simulink model "Gates"  (R2024b)
settings: Solver=FixedStepAuto  StartTime=0  StopTime=1  FixedStep=0.00001  RelTol=1e-3
libraries: spsTriangleGeneratorLib x1
(part 2 of 2)

== system Gates/Subsystem5/Adder & Logic Module/Subsystem6 ==
  Carry In : Inport
  = So far : Inport  Port=2
  A>B Prev : Inport  Port=3
  B : Inport  Port=4
  A : Inport  Port=5
  Subtract : Inport  Port=6
  AND : Logic  IconShape=distinctive  AllPortsSameDT=off  OutDataTypeStr=boolean
  AND1 : Logic  IconShape=distinctive  AllPortsSameDT=off  OutDataTypeStr=boolean
  AND2 : Logic  IconShape=distinctive  AllPortsSameDT=off  OutDataTypeStr=boolean
  AND3 : Logic  Inputs=3  IconShape=distinctive  AllPortsSameDT=off  OutDataTypeStr=boolean
  Mux : Mux  Inputs=6
  NOT : Logic  Operator=NOT  IconShape=distinctive  AllPortsSameDT=off  OutDataTypeStr=boolean
  NOT1 : Logic  Operator=NOT  IconShape=distinctive  AllPortsSameDT=off  OutDataTypeStr=boolean
  NOT2 : Logic  Operator=NOT  IconShape=distinctive  AllPortsSameDT=off  OutDataTypeStr=boolean
  OR : Logic  Operator=OR  IconShape=distinctive  AllPortsSameDT=off  OutDataTypeStr=boolean
  OR1 : Logic  Operator=OR  IconShape=distinctive  AllPortsSameDT=off  OutDataTypeStr=boolean
  OR2 : Logic  Operator=OR  IconShape=distinctive  AllPortsSameDT=off  OutDataTypeStr=boolean
  XOR : Logic  Operator=XOR  IconShape=distinctive  AllPortsSameDT=off  OutDataTypeStr=boolean
  XOR1 : Logic  Operator=XOR  IconShape=distinctive  AllPortsSameDT=off  OutDataTypeStr=boolean
  XOR2 : Logic  Operator=XOR  IconShape=distinctive  AllPortsSameDT=off  OutDataTypeStr=boolean
  Carry Out : Outport
  = Currently : Outport  Port=2
  A >B Next : Outport  Port=3
  Bus : Outport  Port=4
  wires:
  B/1 -> XOR2/1
  Subtract/1 -> XOR2/2
  AND/1 -> OR/1
  AND1/1 -> Mux/2, OR/2  "AND"
  OR/1 -> Carry Out/1
  XOR2/1 -> AND1/2, NOT2/1, OR2/2, XOR/2
  Carry In/1 -> XOR1/2, AND/2
  XOR1/1 -> Mux/1  "Sum"
  XOR/1 -> Mux/4, AND3/3, NOT1/1, XOR1/1, AND/1  "XOR"
  A>B Prev/1 -> OR1/1
  OR1/1 -> A >B Next/1
  NOT1/1 -> AND2/2
  AND2/1 -> = Currently/1
  AND3/1 -> OR1/2
  A/1 -> NOT/1, OR2/1, AND1/1, XOR/1, AND3/2
  = So far/1 -> AND2/1, AND3/1
  OR2/1 -> Mux/3  "OR"
  Mux/1 -> Bus/1
  NOT/1 -> Mux/5  "!A"
  NOT2/1 -> Mux/6  "!B"

== system Gates/Subsystem5/Adder & Logic Module/Subsystem7 ==
  Carry In : Inport
  = So far : Inport  Port=2
  A>B Prev : Inport  Port=3
  B : Inport  Port=4
  A : Inport  Port=5
  Subtract : Inport  Port=6
  AND : Logic  IconShape=distinctive  AllPortsSameDT=off  OutDataTypeStr=boolean
  AND1 : Logic  IconShape=distinctive  AllPortsSameDT=off  OutDataTypeStr=boolean
  AND2 : Logic  IconShape=distinctive  AllPortsSameDT=off  OutDataTypeStr=boolean
  AND3 : Logic  Inputs=3  IconShape=distinctive  AllPortsSameDT=off  OutDataTypeStr=boolean
  Mux : Mux  Inputs=6
  NOT : Logic  Operator=NOT  IconShape=distinctive  AllPortsSameDT=off  OutDataTypeStr=boolean
  NOT1 : Logic  Operator=NOT  IconShape=distinctive  AllPortsSameDT=off  OutDataTypeStr=boolean
  NOT2 : Logic  Operator=NOT  IconShape=distinctive  AllPortsSameDT=off  OutDataTypeStr=boolean
  OR : Logic  Operator=OR  IconShape=distinctive  AllPortsSameDT=off  OutDataTypeStr=boolean
  OR1 : Logic  Operator=OR  IconShape=distinctive  AllPortsSameDT=off  OutDataTypeStr=boolean
  OR2 : Logic  Operator=OR  IconShape=distinctive  AllPortsSameDT=off  OutDataTypeStr=boolean
  XOR : Logic  Operator=XOR  IconShape=distinctive  AllPortsSameDT=off  OutDataTypeStr=boolean
  XOR1 : Logic  Operator=XOR  IconShape=distinctive  AllPortsSameDT=off  OutDataTypeStr=boolean
  XOR2 : Logic  Operator=XOR  IconShape=distinctive  AllPortsSameDT=off  OutDataTypeStr=boolean
  Carry Out : Outport
  = Currently : Outport  Port=2
  A >B Next : Outport  Port=3
  Bus : Outport  Port=4
  wires:
  B/1 -> XOR2/1
  Subtract/1 -> XOR2/2
  AND/1 -> OR/1
  AND1/1 -> Mux/2, OR/2  "AND"
  OR/1 -> Carry Out/1
  XOR2/1 -> AND1/2, NOT2/1, OR2/2, XOR/2
  Carry In/1 -> XOR1/2, AND/2
  XOR1/1 -> Mux/1  "Sum"
  XOR/1 -> Mux/4, AND3/3, NOT1/1, XOR1/1, AND/1  "XOR"
  A>B Prev/1 -> OR1/1
  OR1/1 -> A >B Next/1
  NOT1/1 -> AND2/2
  AND2/1 -> = Currently/1
  AND3/1 -> OR1/2
  A/1 -> NOT/1, OR2/1, AND1/1, XOR/1, AND3/2
  = So far/1 -> AND2/1, AND3/1
  OR2/1 -> Mux/3  "OR"
  Mux/1 -> Bus/1
  NOT/1 -> Mux/5  "!A"
  NOT2/1 -> Mux/6  "!B"

== matlab function Gates/Subsystem5/ALU Selector Bus/MATLAB Function7 ==
  data: InputBus input; output output; Selection input
function output =  Enabler(InputBus, Selection)
    % InputBus: A 6-bit bus representing [SUM, AND, OR, XOR, NOTA, NOTB]
    % Selection: An 8-bit bus where only one bit is active at a time
    % Output: A single bit based on the selected input or shift operation
    
    % Initialize the output as double
    output = 0.0;
    
    % Convert all inputs to double
    SUM_bus = double(InputBus(1));
    
    % Check which selection bit is active and assign the corresponding input
    if Selection(1) == 1
        output = double(InputBus(1)); % SUM
    elseif Selection(2) == 1
        output = double(InputBus(2)); % AND
    elseif Selection(3) == 1
        output = double(InputBus(3)); % OR
    elseif Selection(4) == 1
        output = double(InputBus(4)); % XOR
    elseif Selection(5) == 1
        output = double(InputBus(5)); % NOTA
    elseif Selection(6) == 1
        output = double(InputBus(6)); % NOTB
    elseif Selection(7) == 1
        % Shift right operation on SUM bus
        output = double(bitshift(SUM_bus, -1));
    elseif Selection(8) == 1
        % Shift left operation on SUM bus
        output = double(bitshift(SUM_bus, 1));
    else
        % Default case
        output = 0.0;
    end
end

== matlab function Gates/Subsystem5/ALU Selector Bus/MATLAB Function8 ==
  data: InputBus input; output output; Selection input
function output =  Enabler(InputBus, Selection)
    % InputBus: A 6-bit bus representing [SUM, AND, OR, XOR, NOTA, NOTB]
    % Selection: An 8-bit bus where only one bit is active at a time
    % Output: A single bit based on the selected input or shift operation
    
    % Initialize the output as double
    output = 0.0;
    
    % Convert all inputs to double
    SUM_bus = double(InputBus(1));
    
    % Check which selection bit is active and assign the corresponding input
    if Selection(1) == 1
        output = double(InputBus(1)); % SUM
    elseif Selection(2) == 1
        output = double(InputBus(2)); % AND
    elseif Selection(3) == 1
        output = double(InputBus(3)); % OR
    elseif Selection(4) == 1
        output = double(InputBus(4)); % XOR
    elseif Selection(5) == 1
        output = double(InputBus(5)); % NOTA
    elseif Selection(6) == 1
        output = double(InputBus(6)); % NOTB
    elseif Selection(7) == 1
        % Shift right operation on SUM bus
        output = double(bitshift(SUM_bus, -1));
    elseif Selection(8) == 1
        % Shift left operation on SUM bus
        output = double(bitshift(SUM_bus, 1));
    else
        % Default case
        output = 0.0;
    end
end

== matlab function Gates/Subsystem5/ALU Selector Bus/MATLAB Function6 ==
  data: InputBus input; output output; Selection input
function output =  Enabler(InputBus, Selection)
    % InputBus: A 6-bit bus representing [SUM, AND, OR, XOR, NOTA, NOTB]
    % Selection: An 8-bit bus where only one bit is active at a time
    % Output: A single bit based on the selected input or shift operation
    
    % Initialize the output as double
    output = 0.0;
    
    % Convert all inputs to double
    SUM_bus = double(InputBus(1));
    
    % Check which selection bit is active and assign the corresponding input
    if Selection(1) == 1
        output = double(InputBus(1)); % SUM
    elseif Selection(2) == 1
        output = double(InputBus(2)); % AND
    elseif Selection(3) == 1
        output = double(InputBus(3)); % OR
    elseif Selection(4) == 1
        output = double(InputBus(4)); % XOR
    elseif Selection(5) == 1
        output = double(InputBus(5)); % NOTA
    elseif Selection(6) == 1
        output = double(InputBus(6)); % NOTB
    elseif Selection(7) == 1
        % Shift right operation on SUM bus
        output = double(bitshift(SUM_bus, -1));
    elseif Selection(8) == 1
        % Shift left operation on SUM bus
        output = double(bitshift(SUM_bus, 1));
    else
        % Default case
        output = 0.0;
    end
end

== matlab function Gates/Subsystem5/Adder & Logic Module/MATLAB Function1 ==
  data: Binary input; Decimal output
function Decimal = fcn(Binary)
    % Ensure the input is an 8-bit signal
    assert(length(Binary) == 8, 'Input must be an 8-bit binary signal');
    % Convert the logical array (true/false) to a double array (1/0)
    Binary = double(Binary);
    % Calculate the decimal value
    Decimal = 0;
    for i = 1:8
        Decimal = Decimal + Binary(i) * 2^(8 - i);
    end
end

== matlab function Gates/Subsystem5/Adder & Logic Module/MATLAB Function3 ==
  data: Binary input; Decimal output
function Decimal = fcn(Binary)
    % Ensure the input is an 8-bit signal
    assert(length(Binary) == 8, 'Input must be an 8-bit binary signal');
    % Convert the logical array (true/false) to a double array (1/0)
    Binary = double(Binary);
    % Calculate the decimal value
    Decimal = 0;
    for i = 1:8
        Decimal = Decimal + Binary(i) * 2^(8 - i);
    end
end

== matlab function Gates/MATLAB Function3 ==
  data: number input; a output; b output; c output; d output; e output; f output; g output; h output; Signed output
function [a, b, c, d, e, f, g, h, Signed] = NumToBin(number)
    % Initialise the Signed output
    Signed = false;

    % Ensure the input is within the valid range for unsigned numbers (0 to 255)
    if number < 0
        % For signed mode, enable Signed flag and check if the number is >= -128
        Signed = true;
        if number < -128
            % If below -128, set all outputs to 0
            [a, b, c, d, e, f, g, h] = deal(false, false, false, false, false, false, false, false);
            return;
        else
            % Convert the number to 2's complement representation
            number = 256 + number; % Adjust to positive equivalent for 2's complement
        end
    elseif number > 255
        % If outside the unsigned range, set all outputs to 0
        [a, b, c, d, e, f, g, h] = deal(false, false, false, false, false, false, false, false);
        return;
    end

    % Convert the number to an 8-bit binary using manual calculation
    a = logical(mod(floor(number / 128), 2));
    b = logical(mod(floor(number / 64), 2));
    c = logical(mod(floor(number / 32), 2));
    d = logical(mod(floor(number / 16), 2));
    e = logical(mod(floor(number / 8), 2));
    f = logical(mod(floor(number / 4), 2));
    g = logical(mod(floor(number / 2), 2));
    h = logical(mod(number, 2));
end

== matlab function Gates/Subsystem5/ALU Selector Bus/MATLAB Function1 ==
  data: InputBus input; output output; Selection input
function output =  Enabler(InputBus, Selection)
    % InputBus: A 6-bit bus representing [SUM, AND, OR, XOR, NOTA, NOTB]
    % Selection: An 8-bit bus where only one bit is active at a time
    % Output: A single bit based on the selected input or shift operation
    
    % Initialize the output as double
    output = 0.0;
    
    % Convert all inputs to double
    SUM_bus = double(InputBus(1));
    
    % Check which selection bit is active and assign the corresponding input
    if Selection(1) == 1
        output = double(InputBus(1)); % SUM
    elseif Selection(2) == 1
        output = double(InputBus(2)); % AND
    elseif Selection(3) == 1
        output = double(InputBus(3)); % OR
    elseif Selection(4) == 1
        output = double(InputBus(4)); % XOR
    elseif Selection(5) == 1
        output = double(InputBus(5)); % NOTA
    elseif Selection(6) == 1
        output = double(InputBus(6)); % NOTB
    elseif Selection(7) == 1
        % Shift right operation on SUM bus
        output = double(bitshift(SUM_bus, -1));
    elseif Selection(8) == 1
        % Shift left operation on SUM bus
        output = double(bitshift(SUM_bus, 1));
    else
        % Default case
        output = 0.0;
    end
end

== matlab function Gates/MATLAB Function1 ==
  data: number input; a output; b output; c output; d output; e output; f output; g output; h output; Signed output
function [a, b, c, d, e, f, g, h, Signed] = NumToBin(number)
    % Initialise the Signed output
    Signed = false;

    % Ensure the input is within the valid range for unsigned numbers (0 to 255)
    if number < 0
        % For signed mode, enable Signed flag and check if the number is >= -128
        Signed = true;
        if number < -128
            % If below -128, set all outputs to 0
            [a, b, c, d, e, f, g, h] = deal(false, false, false, false, false, false, false, false);
            return;
        else
            % Convert the number to 2's complement representation
            number = 256 + number; % Adjust to positive equivalent for 2's complement
        end
    elseif number > 255
        % If outside the unsigned range, set all outputs to 0
        [a, b, c, d, e, f, g, h] = deal(false, false, false, false, false, false, false, false);
        return;
    end

    % Convert the number to an 8-bit binary using manual calculation
    a = logical(mod(floor(number / 128), 2));
    b = logical(mod(floor(number / 64), 2));
    c = logical(mod(floor(number / 32), 2));
    d = logical(mod(floor(number / 16), 2));
    e = logical(mod(floor(number / 8), 2));
    f = logical(mod(floor(number / 4), 2));
    g = logical(mod(floor(number / 2), 2));
    h = logical(mod(number, 2));
end

== matlab function Gates/MATLAB Function4 ==
  data: Bin input; Dec output; SM input
function Dec = BinToNum(Bin, SM)
    % Ensure the input is an 8-bit signal
    assert(length(Bin) == 8, 'Input must be an 8-bit binary signal');
    
    % Convert the logical array (true/false) to a double array (1/0)
    Bin = double(Bin);
    
    % Calculate the decimal value
    Dec = 0;
    for i = 1:8
        Dec = Dec + Bin(i) * 2^(8 - i);
    end
    
    % If signed mode is enabled, convert to signed integer using 2's complement
    if SM
        if Bin(1) == 1  % Check if the most significant bit (MSB) is 1 (negative number)
            Dec = Dec - 256;
        end
    end
end

== matlab function Gates/Subsystem5/ALU Selector Bus/MATLAB Function2 ==
  data: InputBus input; output output; Selection input
function output =  Enabler(InputBus, Selection)
    % InputBus: A 6-bit bus representing [SUM, AND, OR, XOR, NOTA, NOTB]
    % Selection: An 8-bit bus where only one bit is active at a time
    % Output: A single bit based on the selected input or shift operation
    
    % Initialize the output as double
    output = 0.0;
    
    % Convert all inputs to double
    SUM_bus = double(InputBus(1));
    
    % Check which selection bit is active and assign the corresponding input
    if Selection(1) == 1
        output = double(InputBus(1)); % SUM
    elseif Selection(2) == 1
        output = double(InputBus(2)); % AND
    elseif Selection(3) == 1
        output = double(InputBus(3)); % OR
    elseif Selection(4) == 1
        output = double(InputBus(4)); % XOR
    elseif Selection(5) == 1
        output = double(InputBus(5)); % NOTA
    elseif Selection(6) == 1
        output = double(InputBus(6)); % NOTB
    elseif Selection(7) == 1
        % Shift right operation on SUM bus
        output = double(bitshift(SUM_bus, -1));
    elseif Selection(8) == 1
        % Shift left operation on SUM bus
        output = double(bitshift(SUM_bus, 1));
    else
        % Default case
        output = 0.0;
    end
end

== matlab function Gates/MATLAB Function2 ==
  data: Bin input; Dec output; SM input
function Dec = BinToNum(Bin, SM)
    % Ensure the input is an 8-bit signal
    assert(length(Bin) == 8, 'Input must be an 8-bit binary signal');
    
    % Convert the logical array (true/false) to a double array (1/0)
    Bin = double(Bin);
    
    % Calculate the decimal value
    Dec = 0;
    for i = 1:8
        Dec = Dec + Bin(i) * 2^(8 - i);
    end
    
    % If signed mode is enabled, convert to signed integer using 2's complement
    if SM
        if Bin(1) == 1  % Check if the most significant bit (MSB) is 1 (negative number)
            Dec = Dec - 256;
        end
    end
end

== matlab function Gates/Subsystem5/ALU Selector Bus/MATLAB Function3 ==
  data: InputBus input; output output; Selection input
function output =  Enabler(InputBus, Selection)
    % InputBus: A 6-bit bus representing [SUM, AND, OR, XOR, NOTA, NOTB]
    % Selection: An 8-bit bus where only one bit is active at a time
    % Output: A single bit based on the selected input or shift operation
    
    % Initialize the output as double
    output = 0.0;
    
    % Convert all inputs to double
    SUM_bus = double(InputBus(1));
    
    % Check which selection bit is active and assign the corresponding input
    if Selection(1) == 1
        output = double(InputBus(1)); % SUM
    elseif Selection(2) == 1
        output = double(InputBus(2)); % AND
    elseif Selection(3) == 1
        output = double(InputBus(3)); % OR
    elseif Selection(4) == 1
        output = double(InputBus(4)); % XOR
    elseif Selection(5) == 1
        output = double(InputBus(5)); % NOTA
    elseif Selection(6) == 1
        output = double(InputBus(6)); % NOTB
    elseif Selection(7) == 1
        % Shift right operation on SUM bus
        output = double(bitshift(SUM_bus, -1));
    elseif Selection(8) == 1
        % Shift left operation on SUM bus
        output = double(bitshift(SUM_bus, 1));
    else
        % Default case
        output = 0.0;
    end
end

== matlab function Gates/Subsystem5/ALU Selector Bus/MATLAB Function4 ==
  data: InputBus input; output output; Selection input
function output =  Enabler(InputBus, Selection)
    % InputBus: A 6-bit bus representing [SUM, AND, OR, XOR, NOTA, NOTB]
    % Selection: An 8-bit bus where only one bit is active at a time
    % Output: A single bit based on the selected input or shift operation
    
    % Initialize the output as double
    output = 0.0;
    
    % Convert all inputs to double
    SUM_bus = double(InputBus(1));
    
    % Check which selection bit is active and assign the corresponding input
    if Selection(1) == 1
        output = double(InputBus(1)); % SUM
    elseif Selection(2) == 1
        output = double(InputBus(2)); % AND
    elseif Selection(3) == 1
        output = double(InputBus(3)); % OR
    elseif Selection(4) == 1
        output = double(InputBus(4)); % XOR
    elseif Selection(5) == 1
        output = double(InputBus(5)); % NOTA
    elseif Selection(6) == 1
        output = double(InputBus(6)); % NOTB
    elseif Selection(7) == 1
        % Shift right operation on SUM bus
        output = double(bitshift(SUM_bus, -1));
    elseif Selection(8) == 1
        % Shift left operation on SUM bus
        output = double(bitshift(SUM_bus, 1));
    else
        % Default case
        output = 0.0;
    end
end

== matlab function Gates/Subsystem5/ALU Selector Bus/MATLAB Function5 ==
  data: InputBus input; output output; Selection input
function output =  Enabler(InputBus, Selection)
    % InputBus: A 6-bit bus representing [SUM, AND, OR, XOR, NOTA, NOTB]
    % Selection: An 8-bit bus where only one bit is active at a time
    % Output: A single bit based on the selected input or shift operation
    
    % Initialize the output as double
    output = 0.0;
    
    % Convert all inputs to double
    SUM_bus = double(InputBus(1));
    
    % Check which selection bit is active and assign the corresponding input
    if Selection(1) == 1
        output = double(InputBus(1)); % SUM
    elseif Selection(2) == 1
        output = double(InputBus(2)); % AND
    elseif Selection(3) == 1
        output = double(InputBus(3)); % OR
    elseif Selection(4) == 1
        output = double(InputBus(4)); % XOR
    elseif Selection(5) == 1
        output = double(InputBus(5)); % NOTA
    elseif Selection(6) == 1
        output = double(InputBus(6)); % NOTB
    elseif Selection(7) == 1
        % Shift right operation on SUM bus
        output = double(bitshift(SUM_bus, -1));
    elseif Selection(8) == 1
        % Shift left operation on SUM bus
        output = double(bitshift(SUM_bus, 1));
    else
        % Default case
        output = 0.0;
    end
end
